simulink model "EE382LastLab"  (R2016a)
settings: Solver=VariableStepAuto  StartTime=0.0  StopTime=4  RelTol=1e-3
libraries: commsrccod2 x2, dspquant2 x2
settings Model: Creator=Tryrant  LastModifiedBy=Tryrant

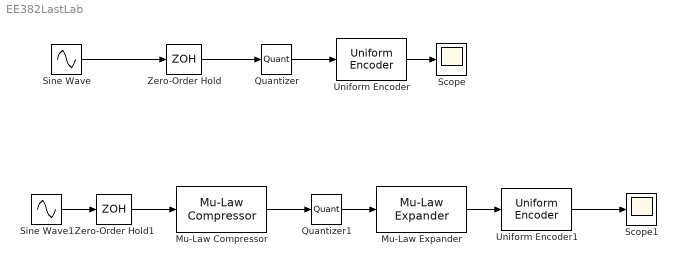
== system EE382LastLab ==
  Mu-Law Compressor : commsrccod2/Mu-Law Compressor  mu=100  V=1
  Mu-Law Expander : commsrccod2/Mu-Law Expander  mu=100  V=1
  Quantizer : Quantizer
  Quantizer1 : Quantizer
  Scope : Scope
  Scope1 : Scope
  Sine Wave : Sin  Frequency=1000  SampleTime=0
  Sine Wave1 : Sin  Frequency=1000  SampleTime=0
  Uniform Encoder : dspquant2/Uniform Encoder  peak=1  bits=32  otype=Unsigned integer
  Uniform Encoder1 : dspquant2/Uniform Encoder  peak=1  bits=32  otype=Unsigned integer
  Zero-Order Hold : ZeroOrderHold  SampleTime=1/100000
  Zero-Order Hold1 : ZeroOrderHold  SampleTime=1/100000
  wires:
  Uniform Encoder/1 -> Scope/1
  Sine Wave/1 -> Zero-Order Hold/1
  Zero-Order Hold/1 -> Quantizer/1
  Quantizer/1 -> Uniform Encoder/1
  Sine Wave1/1 -> Zero-Order Hold1/1
  Zero-Order Hold1/1 -> Mu-Law Compressor/1
  Quantizer1/1 -> Mu-Law Expander/1
  Mu-Law Compressor/1 -> Quantizer1/1
  Mu-Law Expander/1 -> Uniform Encoder1/1
  Uniform Encoder1/1 -> Scope1/1
